simulink subsystem "DE"  (R2024a)
settings: Solver=VariableStepAuto  StartTime=0.0  StopTime=10.0  RelTol=1e-3
settings Model: Creator=prony  LastModifiedBy=prony

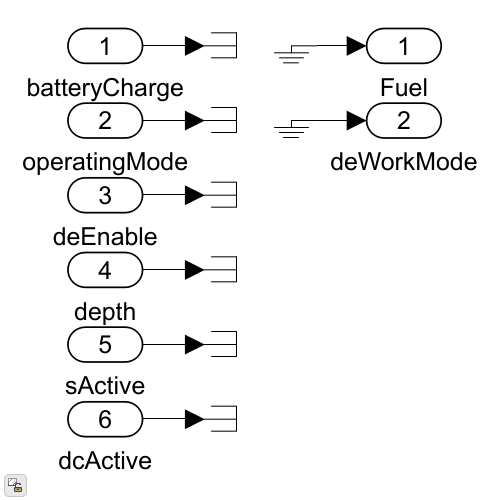
[thumbnail: Simulink's stored preview of the top-level diagram]
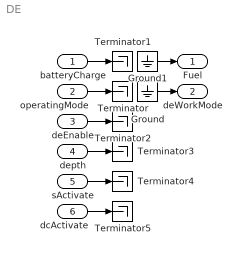
== system DE ==
  batteryCharge : Inport
  operatingMode : Inport  Port=2
  deEnable : Inport  Port=3
  depth : Inport  Port=4
  sActivate : Inport  Port=5
  dcActivate : Inport  Port=6
  Ground : Ground
  Ground1 : Ground
  Terminator{,1..5} (6 alike) : Terminator
  Fuel : Outport
  deWorkMode : Outport  Port=2
  wires:
  Ground/1 -> deWorkMode/1
  operatingMode/1 -> Terminator/1
  batteryCharge/1 -> Terminator1/1
  dcActivate/1 -> Terminator5/1
  sActivate/1 -> Terminator4/1
  depth/1 -> Terminator3/1
  deEnable/1 -> Terminator2/1
  Ground1/1 -> Fuel/1
